simulink model "Teste_Boost"  (R2015a)
settings: Solver=ode45  StartTime=0.0  StopTime=0.05  RelTol=1e-3
libraries: powerlib x13, AvgModels x1, powerlib_meascontrol x1, simulink x1
settings Model: CovSFcnEnable=off  Creator=lgalotto  LastModifiedBy=lgalo
settings DebuggingCC: SolverPrmCheckMsg=warning  UnconnectedInputMsg=none  UnconnectedOutputMsg=none  UnconnectedLineMsg=none

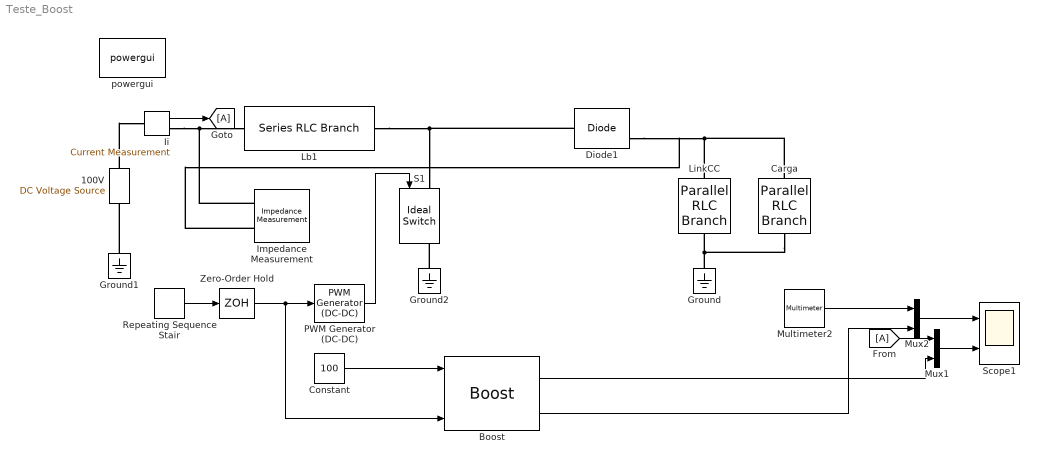
== system Teste_Boost ==
  100V : powerlib/Electrical Sources/DC Voltage Source  Amplitude=100  Measurements=None
  Boost : AvgModels/Conversores Eletrônicos de Potência/Boost  L=280e-6  RL=0.1  C=100e-6  Edit_carga=50  Vini=200  Iini=0  Fs=60000  Vdon=0.8  Rdon=0.001  Vson=0  Rdson=0.001
  Carga : powerlib/Elements/Parallel RLC Branch  LConnTagsString=a  RConnTagsString=__new0  BranchType=R  Resistance=50  Inductance=1e-3  SetiL0=off  InitialCurrent=0  Capacitance=100e-6  Setx0=off  InitialVoltage=0  Measurements=Branch voltage
  Constant : Constant  Value=100
  Diode1 : powerlib/Power Electronics/Diode  Ron=0.001  Lon=0  Vf=0.8  IC=0  UseSnubber=off  Rs=500  Cs=250e-9  Measurements=on
  Ground : powerlib/Elements/Ground  LConnTagsString=a
  Ground1 : powerlib/Elements/Ground  LConnTagsString=a
  Ground2 : powerlib/Elements/Ground  LConnTagsString=a
  Ii : powerlib/Measurements/Current Measurement  PhasorSimulation=off  OutputType=Complex  PSBequivalent=0
  Impedance Measurement : powerlib/Measurements/Impedance Measurement  LConnTagsString=+|-  Factor=1
  Lb1 : powerlib/Elements/Series RLC Branch  LConnTagsString=__new0  RConnTagsString=__new0  BranchType=RL  Resistance=0.1  Inductance=280e-6  SetiL0=off  InitialCurrent=1  Capacitance=1e-6  Setx0=off  InitialVoltage=0  Measurements=Branch current
  LinkCC : powerlib/Elements/Parallel RLC Branch  LConnTagsString=a  RConnTagsString=__new0  BranchType=C  Resistance=10e3  Inductance=1e-3  SetiL0=off  InitialCurrent=0  Capacitance=100e-6  Setx0=on  InitialVoltage=200  Measurements=Branch voltage
  Multimeter2 : powerlib/Measurements/Multimeter  PhasorSimulation=off  OutputType=Complex  sel=2  L=3  Gain=1  yselected={'Ub: LinkCC'};  PSBOutputType=1  PSBequivalent=0  AxesSetting=[0,0.1,-100,100]  Display=0  SavedBlockNames=-11
  Mux1 : Mux  Inputs=2
  Mux2 : Mux  Inputs=2
  PWM Generator (DC-DC) : powerlib_meascontrol/Pulse & Signal Generators/PWM Generator (DC-DC)  Fsw=60000  Ts=0
  Repeating Sequence Stair : simulink/Sources/Repeating Sequence Stair  OutValues=[0.2 0.4 0.6 0.8 0.6 0.2].'  tsamp=0.01  OutMin=[]  OutMax=[]  OutDataTypeStr=double  OutputDataTypeScalingMode=double  OutDataType=fixdt(0,8)  ConRadixGroup=Best Precision: Vector-wise  OutScaling=2^-12
  S1 : powerlib/Power Electronics/Ideal Switch  Ron=0.001  Lon=0  IC=0  Rs=1e5  Cs=inf  Measurements=on
  Scope1 : Scope  NumInputPorts=2
      settings: TimeRange=0.05  YMin=100~-20  YMax=600~160
  Zero-Order Hold : ZeroOrderHold  SampleTime=0.01
  powergui : powerlib/powergui  Priority=1  SimulationMode=Continuous  SolverType=Tustin  SampleTime=50e-6  frequency=60  SPID=on  DisableSnubberDevices=off  DisableRonSwitches=off  DisableVfSwitches=off  SwTol=0  DisplayEquations=off  Interpol=off  methode=off  Ts=0  FunctionMessages=off  echomessages=off  HookPort=off  EnableUseOfTLC=off  x0status=blocks  frequencyindice=0  Pbase=100e6  ErrMax=1e-4  Iterations=50  UnitsV=kV  UnitsW=MW  buscounter=0  RestoreLinks=warning  ResistiveCurrentMeasurement=off  Frange=[0:2:500]  Ylog=off  Xlog=on  ShowGrid=off  save=off  variable=ZData  structure=0  ZoomFFT=off  StartTime=0.0  cycles=1  DisplayStyle=1  fundamental=60  FreqAxis=off  MaxFrequency=1000  frequencyindicesteady=1  RmsSteady=1  display=off
  wires:
  PWM Generator (DC-DC)/1 -> S1/1
  Zero-Order Hold/1 -> Boost/3, PWM Generator (DC-DC)/1
  [A] -> Mux1/1
  Ii/1 -> [A]
  Constant/1 -> Boost/1
  Multimeter2/1 -> Mux2/1
  Boost/2 -> Mux2/2
  Boost/1 -> Mux1/2
  Mux1/1 -> Scope1/2
  Mux2/1 -> Scope1/1
  Repeating Sequence Stair/1 -> Zero-Order Hold/1
  connections:
  Impedance Measurement/LConn1 -- Ii/RConn1 -- Lb1/LConn1
  Lb1/RConn1 -- Diode1/LConn1 -- S1/LConn1
  Impedance Measurement/LConn2 -- Diode1/RConn1 -- Carga/LConn1 -- LinkCC/LConn1
  Ground1/LConn1 -- 100V/LConn1
  Ground/LConn1 -- Carga/RConn1 -- LinkCC/RConn1
  Ground2/LConn1 -- S1/RConn1
  100V/RConn1 -- Ii/LConn1
